simulink model "entrelace"  (R2021b)
settings: Solver=VariableStepAuto  StartTime=0.0  StopTime=0.013  RelTol=1e-3
libraries: spsDiodeLib x5, spsSeriesRLCBranchLib x3, spsCurrentMeasurementLib x2, spsLinearTransformerLib x2, spsMosfetLib x2, spsVoltageMeasurementLib x2, spsDCVoltageSourceLib x1, spspowerguiLib x1
settings Model: Creator=mouht  LastModifiedBy=mouht

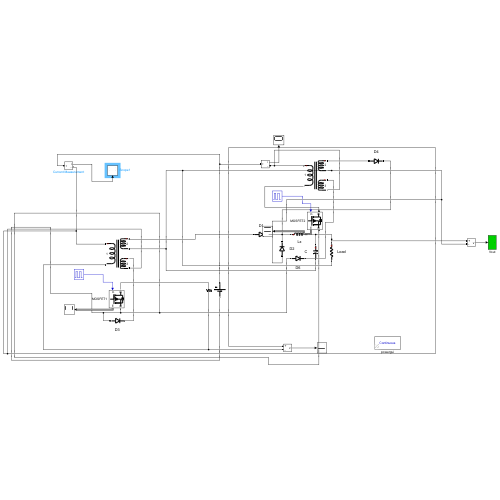
[thumbnail: Simulink's stored preview of the top-level diagram]
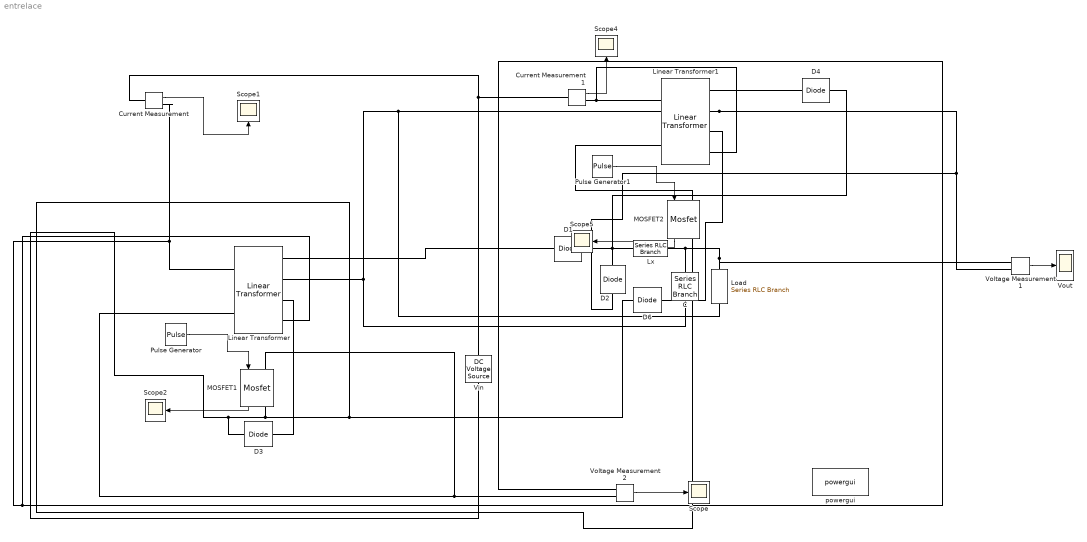
== system entrelace ==
  C : spsSeriesRLCBranchLib/Series RLC Branch  LConnTagsString=__new0  RConnTagsString=__new0  BranchType=C  Resistance=1e-4  Inductance=200e-6  SetiL0=off  InitialCurrent=0  Capacitance=100e-6  Setx0=off  InitialVoltage=0  Measurements=None
  Current Measurement : spsCurrentMeasurementLib/Current Measurement  PhasorSimulation=off  OutputType=Complex  PSBequivalent=0
  Current Measurement1 : spsCurrentMeasurementLib/Current Measurement  PhasorSimulation=off  OutputType=Complex  PSBequivalent=0
  D{1..4,6} (5 alike) : spsDiodeLib/Diode  Ron=1e-3  Lon=0  Vf=0  IC=0  UseSnubber=off  Rs=inf  Cs=0  Measurements=off
  Linear Transformer : spsLinearTransformerLib/Linear Transformer  UNITS=SI  NominalPower=[ 25 100e3 ]  winding1=[24 0 0]  winding2=[16 0 0]  ThreeWindings=on  winding3=[24 0 0]  RmLm=[inf 10e-3]  Measurements=Magnetization current  DataType=on
  Linear Transformer1 : spsLinearTransformerLib/Linear Transformer  UNITS=SI  NominalPower=[ 25 100e3 ]  winding1=[24 0 0]  winding2=[16 0 0]  ThreeWindings=on  winding3=[24 0 0]  RmLm=[inf 10e-3]  Measurements=Magnetization current  DataType=on
  Load : spsSeriesRLCBranchLib/Series RLC Branch  LConnTagsString=__new0  RConnTagsString=__new0  BranchType=R  Resistance=10  Inductance=200e-6  SetiL0=off  InitialCurrent=0  Capacitance=400e-6  Setx0=off  InitialVoltage=0  Measurements=Branch current
  Lx : spsSeriesRLCBranchLib/Series RLC Branch  LConnTagsString=__new0  RConnTagsString=__new0  BranchType=L  Resistance=10  Inductance=400e-6  SetiL0=off  InitialCurrent=0  Capacitance=400e-6  Setx0=off  InitialVoltage=0  Measurements=Branch current
  MOSFET1 : spsMosfetLib/Mosfet  Ron=1e-6  Lon=0  Rd=1e-3  Vfd=0  IC=0  Rs=1e6  Cs=inf  Measurements=on
  MOSFET2 : spsMosfetLib/Mosfet  Ron=1e-6  Lon=0  Rd=1e-3  Vfd=0  IC=0  Rs=1e6  Cs=inf  Measurements=on
  Pulse Generator : DiscretePulseGenerator  PulseType=Time based  Period=1/35e3  PulseWidth=40
  Pulse Generator1 : DiscretePulseGenerator  PulseType=Time based  Period=1/35e3  PulseWidth=40
  Scope{,1..2,4..5} (5 alike) : Scope
  Vin : spsDCVoltageSourceLib/DC Voltage Source  Amplitude=48  Measurements=None
  Voltage Measurement1 : spsVoltageMeasurementLib/Voltage Measurement  PhasorSimulation=off  OutputType=Complex  PSBequivalent=0
  Voltage Measurement2 : spsVoltageMeasurementLib/Voltage Measurement  PhasorSimulation=off  OutputType=Complex  PSBequivalent=0
  Vout : Scope
  powergui : spspowerguiLib/powergui  Priority=1  SimulationMode=Continuous  SampleTime=50e-6  frequency=60  Iterations=50  frequencyindice=0  Pbase=100e6  ErrMax=1e-4  UnitsV=kV  UnitsW=MW  buscounter=0  FunctionMessages=off  echomessages=off  EnableUseOfTLC=off  CurrentSourceSwitches=off  DisableSnubberDevices=off  DisableRonSwitches=off  DisableVfSwitches=off  DisplayEquations=off  AutomaticDiscreteSolvers=off  SolverType=Tustin/Backward Euler (TBE)  Interpol=off  ExternalGateDelay=off  methode=off  Ts=100  x0status=blocks  SPID=on  SwTol=0  HookPort=off  NonlinearTolerance=1e-4  nMaxIteration=100  ContinueOnMaxIteration=off  RestoreLinks=warning  ResistiveCurrentMeasurement=off  Frange=[0:2:500]  Ylog=off  Xlog=on  ShowGrid=off  save=off  variable=ZData  structure=0  ZoomFFT=off  StartTime=0.0  cycles=1  DisplayStyle=1  fundamental=60  FreqAxis=off  MaxFrequency=1000  frequencyindicesteady=1  RmsSteady=1  display=off
  wires:
  Current Measurement/1 -> Scope1/1
  Voltage Measurement2/1 -> Scope/1
  Pulse Generator/1 -> MOSFET1/1
  Voltage Measurement1/1 -> Vout/1
  MOSFET1/1 -> Scope2/1
  MOSFET2/1 -> Scope5/1
  Pulse Generator1/1 -> MOSFET2/1
  Current Measurement1/1 -> Scope4/1
  connections:
  Current Measurement/RConn1 -- Linear Transformer/LConn1 -- Voltage Measurement2/LConn1 -- Linear Transformer/RConn4
  Load/RConn1 -- Voltage Measurement1/LConn2 -- D2/LConn1 -- Linear Transformer1/RConn2 -- C/RConn1 -- Linear Transformer/RConn2
  MOSFET2/RConn1 -- Vin/LConn1 -- D3/LConn1 -- MOSFET1/RConn1 -- D6/LConn1
  MOSFET1/LConn1 -- Voltage Measurement2/LConn2 -- Linear Transformer/LConn2
  Lx/RConn1 -- Load/LConn1 -- Voltage Measurement1/LConn1 -- C/LConn1
  D2/RConn1 -- D4/RConn1 -- D1/RConn1 -- Lx/LConn1
  Vin/RConn1 -- Current Measurement1/LConn1 -- Current Measurement/LConn1
  D1/LConn1 -- Linear Transformer/RConn1
  D3/RConn1 -- Linear Transformer/RConn3
  Linear Transformer1/LConn2 -- MOSFET2/LConn1
  Linear Transformer1/LConn1 -- Current Measurement1/RConn1 -- Linear Transformer1/RConn4
  D6/RConn1 -- Linear Transformer1/RConn3
  D4/LConn1 -- Linear Transformer1/RConn1
